simulink model "CE141IntroModel3"  (R2014b)
settings: Solver=ode45  StartTime=0.0  StopTime=40  MaxStep=0.1  RelTol=1e-3
settings Model: Creator=Dejan  LastModifiedBy=Dejan
settings DataIOCC: SignalLoggingSaveFormat=ModelDataLogs
settings OptimizationCC: ExpressionDepthLimit=2147483647
settings DebuggingCC: UnderspecifiedInitializationDetection=Classic  MergeDetectMultiDrivingBlocksExec=none  SolverPrmCheckMsg=none  FcnCallInpInsideContextMsg=EnableAllAsWarning  StateNameClashWarn=warning
settings GRTTargetCC: CombineOutputUpdateFcns=off  GRTInterface=on

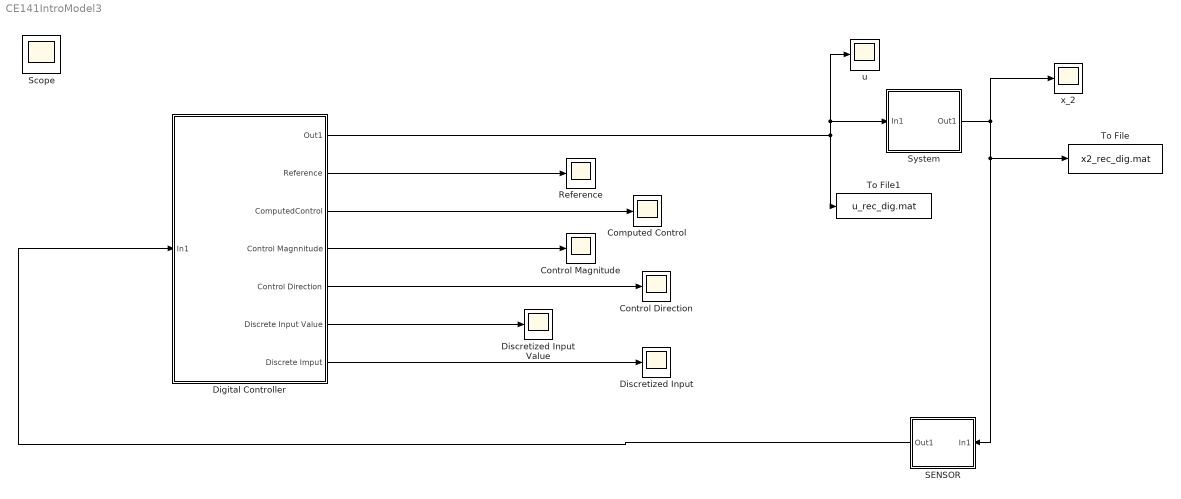
== system CE141IntroModel3 ==
  Computed Control : Scope
      settings: SaveName=ScopeData2
  Control Direction : Scope
      settings: SaveName=ScopeData5
  Control Magnitude : Scope
      settings: SaveName=ScopeData4
  Digital Controller : Subsystem
  Discretized Input : Scope
      settings: SaveName=ScopeData6
  Discretized Input Value : Scope
      settings: SaveName=ScopeData7
  Reference : Scope
      settings: SaveName=ScopeData3
  SENSOR : Subsystem
  System : Subsystem
  To File : ToFile  Filename=x2_rec_dig.mat  MatrixName=x2_rec_dig  SaveFormat=Timeseries
  To File1 : ToFile  Filename=u_rec_dig.mat  MatrixName=u_rec_dig  SaveFormat=Timeseries
  u : Scope
  x_2 : Scope
      settings: TimeRange=4  YMin=-3.65625  YMax=0.3437500000000004
  Scope : Scope
      settings: MaxDataPoints=7500
  wires:
  System/1(Out1) -> x_2/1, SENSOR/1(In1), To File/1
  Digital Controller/1(Out1) -> u/1, System/1(In1), To File1/1
  SENSOR/1(Out1) -> Digital Controller/1(In1)
  Digital Controller/2(Reference) -> Reference/1
  Digital Controller/3(ComputedControl) -> Computed Control/1
  Digital Controller/4(Control Magnnitude) -> Control Magnitude/1
  Digital Controller/5(Control Direction) -> Control Direction/1
  Digital Controller/7(Discrete Imput) -> Discretized Input/1
  Digital Controller/6(Discrete Input Value) -> Discretized Input Value/1

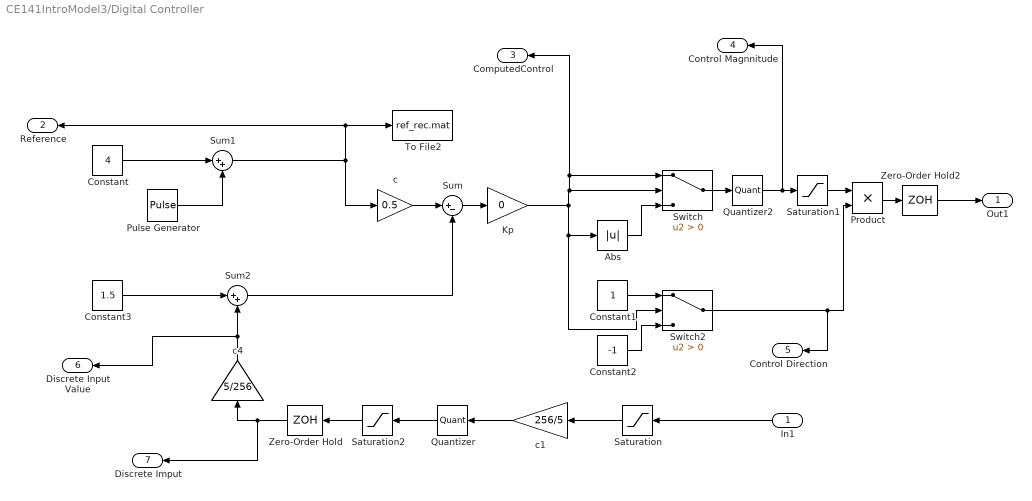
== system CE141IntroModel3/Digital Controller ==
  In1 : Inport
  Abs : Abs
  Constant : Constant  Value=4
  Constant1 : Constant
  Constant2 : Constant  Value=-1
  Constant3 : Constant  Value=1.5
  Kp : Gain  Gain=0
  Product : Product
  Pulse Generator : DiscretePulseGenerator  PulseType=Time based  Amplitude=1.4  Period=10  PulseWidth=50  PhaseDelay=5
  Quantizer : Quantizer
  Quantizer2 : Quantizer  QuantizationInterval=5/255
  Saturation : Saturate  UpperLimit=5  LowerLimit=0
  Saturation1 : Saturate  UpperLimit=5  LowerLimit=0
  Saturation2 : Saturate  UpperLimit=255  LowerLimit=0
  Sum : Sum  Inputs=|+-
  Sum1 : Sum  Inputs=|++
  Sum2 : Sum  Inputs=|++
  Switch : Switch  Criteria=u2 > Threshold
  Switch2 : Switch  Criteria=u2 > Threshold
  To File2 : ToFile  Filename=ref_rec.mat  MatrixName=ref_rec  SaveFormat=Timeseries
  Zero-Order Hold : ZeroOrderHold  SampleTime=0.3
  Zero-Order Hold2 : ZeroOrderHold  SampleTime=0.3
  c : Gain  Gain=0.5
  c1 : Gain  Gain=256/5
  c4 : Gain  Gain=5/256
  Out1 : Outport
  Reference : Outport  Port=2
  ComputedControl : Outport  Port=3
  Control Magnnitude : Outport  Port=4
  Control Direction : Outport  Port=5
  Discrete Input Value : Outport  Port=6
  Discrete Imput : Outport  Port=7
  wires:
  In1/1 -> Saturation/1
  Pulse Generator/1 -> Sum1/2
  Sum/1 -> Kp/1
  Constant/1 -> Sum1/1
  Zero-Order Hold2/1 -> Out1/1
  Quantizer2/1 -> Control Magnnitude/1, Saturation1/1
  Saturation1/1 -> Product/1
  Constant1/1 -> Switch2/1
  Product/1 -> Zero-Order Hold2/1
  Constant2/1 -> Switch2/3
  Switch2/1 -> Control Direction/1, Product/2
  Switch/1 -> Quantizer2/1
  Kp/1 -> Switch/2, ComputedControl/1, Switch/1, Switch2/2, Abs/1
  Abs/1 -> Switch/3
  Sum1/1 -> To File2/1, Reference/1, c/1
  Saturation/1 -> c1/1
  c1/1 -> Quantizer/1
  Quantizer/1 -> Saturation2/1
  Saturation2/1 -> Zero-Order Hold/1
  Constant3/1 -> Sum2/1
  Sum2/1 -> Sum/2
  Zero-Order Hold/1 -> Discrete Imput/1, c4/1
  c4/1 -> Discrete Input Value/1, Sum2/2
  c/1 -> Sum/1

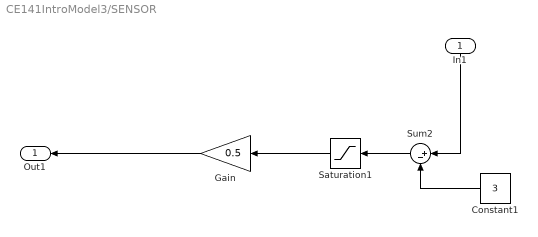
== system CE141IntroModel3/SENSOR ==
  In1 : Inport
  Constant1 : Constant  Value=3
  Gain : Gain  Gain=0.5
  Saturation1 : Saturate  UpperLimit=5  LowerLimit=0
  Sum2 : Sum  Inputs=|+-
  Out1 : Outport
  wires:
  In1/1 -> Sum2/1
  Constant1/1 -> Sum2/2
  Sum2/1 -> Saturation1/1
  Saturation1/1 -> Gain/1
  Gain/1 -> Out1/1

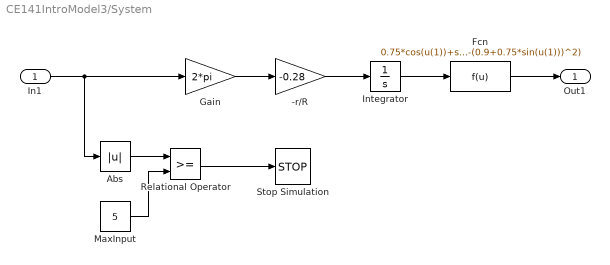
== system CE141IntroModel3/System ==
  In1 : Inport
  -r/R : Gain  Gain=-0.28
  Abs : Abs
  Fcn : Fcn  Expr=0.75*cos(u(1))+sqrt(4.8^2-(0.9+0.75*sin(u(1)))^2)
  Gain : Gain  Gain=2*pi
  Integrator : Integrator  InitialCondition=1
  MaxInput : Constant  Value=5
  Relational Operator : RelationalOperator  OutDataTypeStr=boolean
  Stop Simulation : Stop
  Out1 : Outport
  wires:
  Integrator/1 -> Fcn/1
  Fcn/1 -> Out1/1
  Gain/1 -> -r/R/1
  -r/R/1 -> Integrator/1
  Relational Operator/1 -> Stop Simulation/1
  In1/1 -> Abs/1, Gain/1
  Abs/1 -> Relational Operator/1
  MaxInput/1 -> Relational Operator/2
